simulink model "DinamicSystem"  (R2022b)
settings: Solver=VariableStepAuto  StartTime=0.0  StopTime=10.0  RelTol=1e-3
settings Model: Creator=1NR_Operator_34  LastModifiedBy=1NR_Operator_34
settings SolverCC: AlgebraicLoopSolver=TrustRegion
settings DebuggingCC: UnconnectedInputMsg=warning  UnconnectedOutputMsg=warning  UnconnectedLineMsg=warning  SFMachineParentedDataDiag=warning
settings ModelReferenceCC: EnableRefExpFcnMdlSchedulingChecks=on

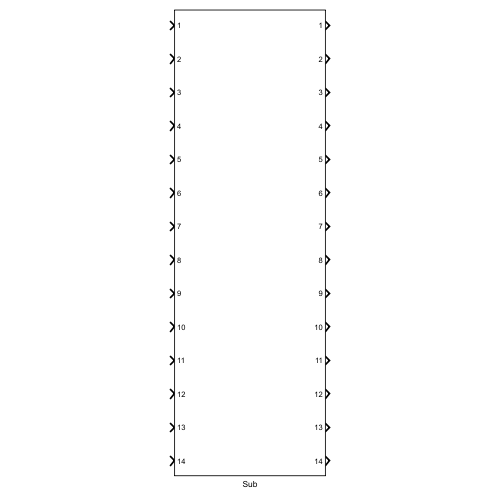
[thumbnail: Simulink's stored preview of the top-level diagram]
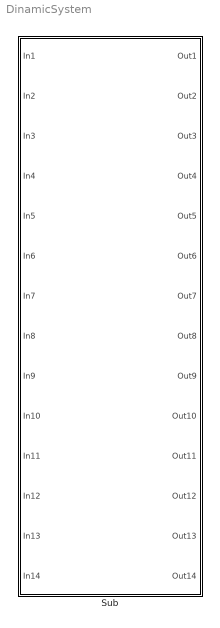
== system DinamicSystem ==
  Sub : Subsystem

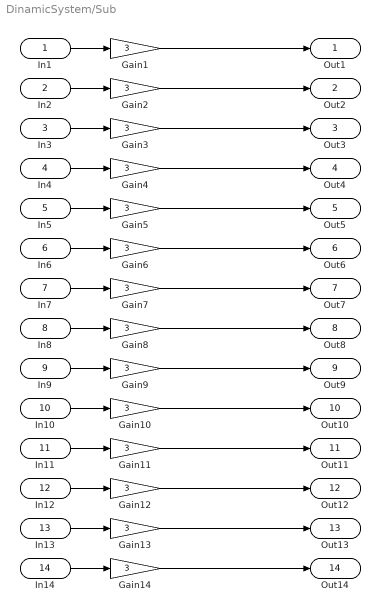
== system DinamicSystem/Sub ==
  In1 : Inport
  In2 : Inport  Port=2
  In3 : Inport  Port=3
  In4 : Inport  Port=4
  In5 : Inport  Port=5
  In6 : Inport  Port=6
  In7 : Inport  Port=7
  In8 : Inport  Port=8
  In9 : Inport  Port=9
  In10 : Inport  Port=10
  In11 : Inport  Port=11
  In12 : Inport  Port=12
  In13 : Inport  Port=13
  In14 : Inport  Port=14
  Gain{1..14} (14 alike) : Gain  Gain=3
  Out1 : Outport
  Out2 : Outport  Port=2
  Out3 : Outport  Port=3
  Out4 : Outport  Port=4
  Out5 : Outport  Port=5
  Out6 : Outport  Port=6
  Out7 : Outport  Port=7
  Out8 : Outport  Port=8
  Out9 : Outport  Port=9
  Out10 : Outport  Port=10
  Out11 : Outport  Port=11
  Out12 : Outport  Port=12
  Out13 : Outport  Port=13
  Out14 : Outport  Port=14
  wires:
  In1/1 -> Gain1/1
  In2/1 -> Gain2/1
  In3/1 -> Gain3/1
  In4/1 -> Gain4/1
  In5/1 -> Gain5/1
  In6/1 -> Gain6/1
  In7/1 -> Gain7/1
  In8/1 -> Gain8/1
  In9/1 -> Gain9/1
  In10/1 -> Gain10/1
  In11/1 -> Gain11/1
  In12/1 -> Gain12/1
  In13/1 -> Gain13/1
  In14/1 -> Gain14/1
  Gain1/1 -> Out1/1
  Gain2/1 -> Out2/1
  Gain3/1 -> Out3/1
  Gain4/1 -> Out4/1
  Gain5/1 -> Out5/1
  Gain6/1 -> Out6/1
  Gain7/1 -> Out7/1
  Gain8/1 -> Out8/1
  Gain9/1 -> Out9/1
  Gain10/1 -> Out10/1
  Gain11/1 -> Out11/1
  Gain12/1 -> Out12/1
  Gain13/1 -> Out13/1
  Gain14/1 -> Out14/1
